simulink model "disturbances"  (R2018b)
settings: Solver=ode45  StartTime=0.0  StopTime=100  RelTol=1e-3
settings Model: Creator=Bashar  LastModifiedBy=Bashar

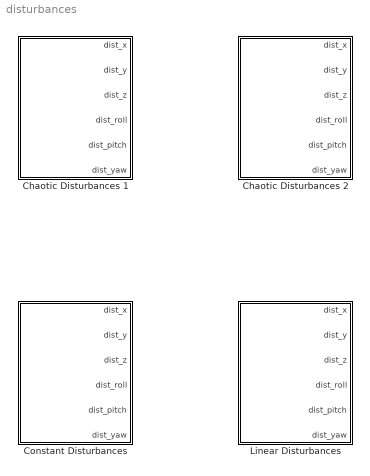
== system disturbances ==
  Chaotic Disturbances 1 : Subsystem
  Chaotic Disturbances 2 : Subsystem
  Constant Disturbances : Subsystem
  Linear Disturbances : Subsystem

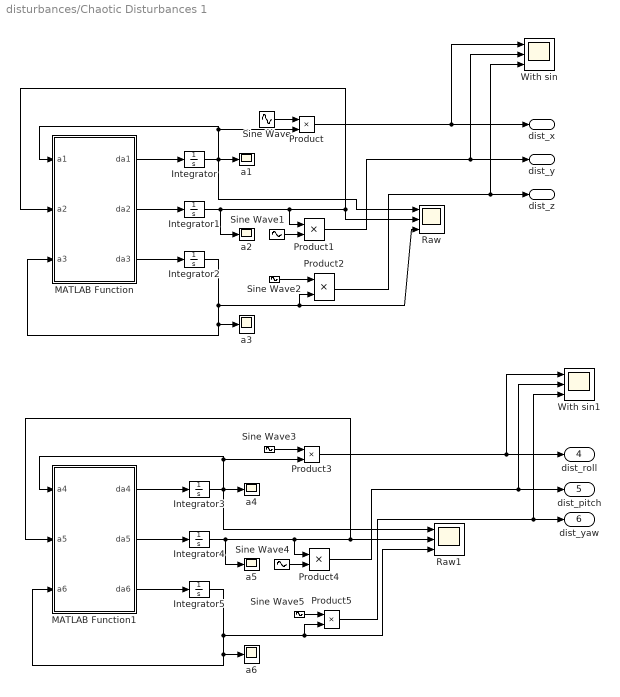
== system disturbances/Chaotic Disturbances 1 ==
  Integrator : Integrator  InitialCondition=-6
  Integrator1 : Integrator  InitialCondition=-5
  Integrator2 : Integrator  InitialCondition=22
  Integrator3 : Integrator  InitialCondition=-10
  Integrator4 : Integrator  InitialCondition=-12
  Integrator5 : Integrator  InitialCondition=24
  MATLAB Function : MATLAB Function  TreatAsAtomicUnit=on
  MATLAB Function1 : MATLAB Function  TreatAsAtomicUnit=on
  Product{,1..5} (6 alike) : Product
  Raw : Scope  NumInputPorts=3
  Raw1 : Scope  NumInputPorts=3
  Sine Wave : Sin  Amplitude=0.01  Frequency=0.5  Phase=-25  SampleTime=0
  Sine Wave1 : Sin  Amplitude=0.01  Frequency=0.5  Phase=-45  SampleTime=0
  Sine Wave2 : Sin  Amplitude=0.01  Frequency=0.5  Phase=-65  SampleTime=0
  Sine Wave3 : Sin  Amplitude=0.01  Frequency=0.5  Phase=-10  SampleTime=0
  Sine Wave4 : Sin  Amplitude=0.01  Frequency=0.5  Phase=-30  SampleTime=0
  Sine Wave5 : Sin  Amplitude=0.01  Frequency=0.5  Phase=-50  SampleTime=0
  With sin : Scope  NumInputPorts=3
  With sin1 : Scope  NumInputPorts=3
  "a1 " : Scope
  a{2..6} (5 alike) : Scope
  dist_x : Outport
  dist_y : Outport  Port=2
  dist_z : Outport  Port=3
  dist_roll : Outport  Port=4
  dist_pitch : Outport  Port=5
  dist_yaw : Outport  Port=6
  wires:
  MATLAB Function1/2(da5) -> Integrator4/1
  Sine Wave3/1 -> Product3/1
  Sine Wave4/1 -> Product4/2
  Product5/1 -> With sin1/3, dist_yaw/1
  Sine Wave5/1 -> Product5/1
  Integrator4/1 -> Product4/1, MATLAB Function1/2(a5), Raw1/2, a5/1
  Integrator/1 -> Raw/1, MATLAB Function/1(a1), Product/2, "a1 "/1
  Sine Wave/1 -> Product/1
  Integrator3/1 -> Raw1/1, MATLAB Function1/1(a4), Product3/2, a4/1
  MATLAB Function/3(da3) -> Integrator2/1
  MATLAB Function1/1(da4) -> Integrator3/1
  Product3/1 -> With sin1/1, dist_roll/1
  MATLAB Function1/3(da6) -> Integrator5/1
  Product4/1 -> With sin1/2, dist_pitch/1
  Integrator1/1 -> Product1/1, MATLAB Function/2(a2), Raw/2, a2/1
  MATLAB Function/2(da2) -> Integrator1/1
  MATLAB Function/1(da1) -> Integrator/1
  Integrator2/1 -> Product2/2, Raw/3, MATLAB Function/3(a3), a3/1
  Sine Wave2/1 -> Product2/1
  Sine Wave1/1 -> Product1/2
  Product2/1 -> With sin/3, dist_z/1
  Product/1 -> With sin/1, dist_x/1
  Product1/1 -> With sin/2, dist_y/1
  Integrator5/1 -> Product5/2, Raw1/3, MATLAB Function1/3(a6), a6/1

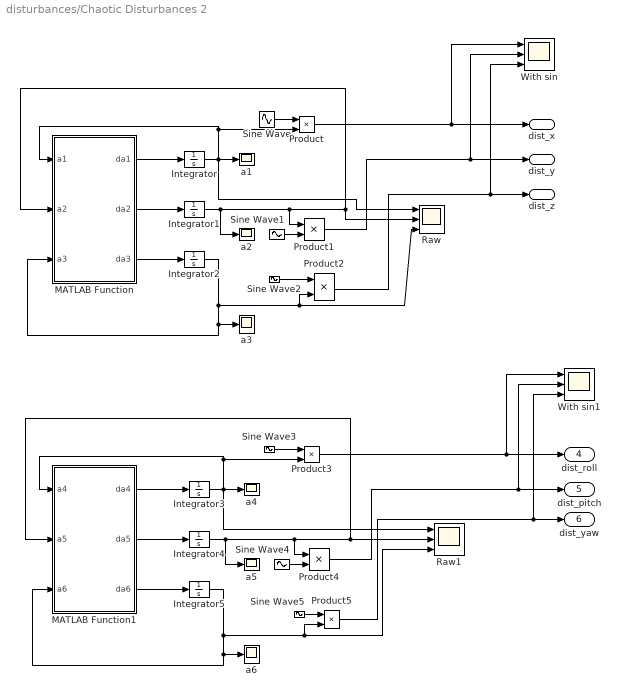
== system disturbances/Chaotic Disturbances 2 ==
  Integrator : Integrator  InitialCondition=-2
  Integrator1 : Integrator  InitialCondition=-8
  Integrator2 : Integrator  InitialCondition=15
  Integrator3 : Integrator  InitialCondition=-4
  Integrator4 : Integrator  InitialCondition=-15
  Integrator5 : Integrator  InitialCondition=20
  MATLAB Function : MATLAB Function  TreatAsAtomicUnit=on
  MATLAB Function1 : MATLAB Function  TreatAsAtomicUnit=on
  Product{,1..5} (6 alike) : Product
  Raw : Scope  NumInputPorts=3
  Raw1 : Scope  NumInputPorts=3
  Sine Wave : Sin  Amplitude=0.01  Frequency=0.5  Phase=-20  SampleTime=0
  Sine Wave1 : Sin  Amplitude=0.01  Frequency=0.5  Phase=-40  SampleTime=0
  Sine Wave2 : Sin  Amplitude=0.01  Frequency=0.5  Phase=-60  SampleTime=0
  Sine Wave3 : Sin  Amplitude=0.01  Frequency=0.5  Phase=-15  SampleTime=0
  Sine Wave4 : Sin  Amplitude=0.01  Frequency=0.5  Phase=-35  SampleTime=0
  Sine Wave5 : Sin  Amplitude=0.01  Frequency=0.5  Phase=-55  SampleTime=0
  With sin : Scope  NumInputPorts=3
  With sin1 : Scope  NumInputPorts=3
  "a1 " : Scope
  a{2..6} (5 alike) : Scope
  dist_x : Outport
  dist_y : Outport  Port=2
  dist_z : Outport  Port=3
  dist_roll : Outport  Port=4
  dist_pitch : Outport  Port=5
  dist_yaw : Outport  Port=6
  wires:
  MATLAB Function1/2(da5) -> Integrator4/1
  Sine Wave3/1 -> Product3/1
  Sine Wave4/1 -> Product4/2
  Product5/1 -> With sin1/3, dist_yaw/1
  Sine Wave5/1 -> Product5/1
  Integrator4/1 -> Product4/1, MATLAB Function1/2(a5), Raw1/2, a5/1
  Integrator/1 -> Raw/1, MATLAB Function/1(a1), Product/2, "a1 "/1
  Sine Wave/1 -> Product/1
  Integrator3/1 -> Raw1/1, MATLAB Function1/1(a4), Product3/2, a4/1
  MATLAB Function/3(da3) -> Integrator2/1
  MATLAB Function1/1(da4) -> Integrator3/1
  Product3/1 -> With sin1/1, dist_roll/1
  MATLAB Function1/3(da6) -> Integrator5/1
  Product4/1 -> With sin1/2, dist_pitch/1
  Integrator1/1 -> Product1/1, MATLAB Function/2(a2), Raw/2, a2/1
  MATLAB Function/2(da2) -> Integrator1/1
  MATLAB Function/1(da1) -> Integrator/1
  Integrator2/1 -> Product2/2, Raw/3, MATLAB Function/3(a3), a3/1
  Sine Wave2/1 -> Product2/1
  Sine Wave1/1 -> Product1/2
  Product2/1 -> With sin/3, dist_z/1
  Product/1 -> With sin/1, dist_x/1
  Product1/1 -> With sin/2, dist_y/1
  Integrator5/1 -> Product5/2, Raw1/3, MATLAB Function1/3(a6), a6/1

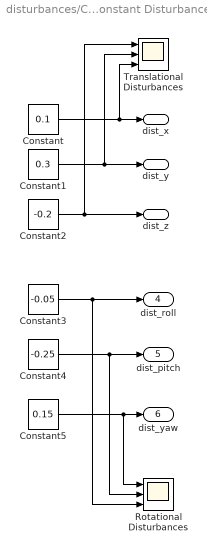
== system disturbances/Constant Disturbances ==
  Constant : Constant  Value=0.1
  Constant1 : Constant  Value=0.3
  Constant2 : Constant  Value=-0.2
  Constant3 : Constant  Value=-0.05
  Constant4 : Constant  Value=-0.25
  Constant5 : Constant  Value=0.15
  Rotational Disturbances : Scope  NumInputPorts=3
  Translational Disturbances : Scope  NumInputPorts=3
  dist_x : Outport
  dist_y : Outport  Port=2
  dist_z : Outport  Port=3
  dist_roll : Outport  Port=4
  dist_pitch : Outport  Port=5
  dist_yaw : Outport  Port=6
  wires:
  Constant/1 -> Translational Disturbances/3, dist_x/1
  Constant1/1 -> Translational Disturbances/2, dist_y/1
  Constant2/1 -> Translational Disturbances/1, dist_z/1
  Constant3/1 -> Rotational Disturbances/3, dist_roll/1
  Constant4/1 -> dist_pitch/1, Rotational Disturbances/2
  Constant5/1 -> Rotational Disturbances/1, dist_yaw/1

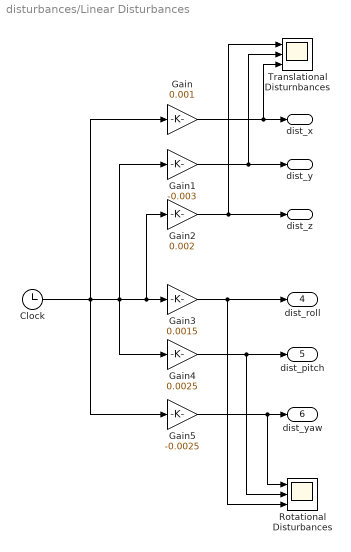
== system disturbances/Linear Disturbances ==
  Clock : Clock
  Gain : Gain  Gain=0.001
  Gain1 : Gain  Gain=-0.003
  Gain2 : Gain  Gain=0.002
  Gain3 : Gain  Gain=0.0015
  Gain4 : Gain  Gain=0.0025
  Gain5 : Gain  Gain=-0.0025
  Rotational Disturbances : Scope  NumInputPorts=3
  Translational Disturnbances : Scope  NumInputPorts=3
  dist_x : Outport
  dist_y : Outport  Port=2
  dist_z : Outport  Port=3
  dist_roll : Outport  Port=4
  dist_pitch : Outport  Port=5
  dist_yaw : Outport  Port=6
  wires:
  Gain/1 -> Translational Disturnbances/3, dist_x/1
  Gain1/1 -> Translational Disturnbances/2, dist_y/1
  Gain2/1 -> Translational Disturnbances/1, dist_z/1
  Gain3/1 -> dist_roll/1, Rotational Disturbances/3
  Gain4/1 -> dist_pitch/1, Rotational Disturbances/2
  Gain5/1 -> Rotational Disturbances/1, dist_yaw/1
  Clock/1 -> Gain2/1, Gain3/1, Gain4/1, Gain1/1, Gain5/1, Gain/1

== matlab function disturbances/Chaotic Disturbances 2/MATLAB Function ==
  data: a1 input; da1 output; a2 input; a3 input; da2 output; da3 output
function [da1, da2, da3] = lorenz_system(a1, a2, a3)
sigma = 10; rho = 28; beta = 8/3;
da1 = 0.1*(sigma*(a2-a1));
da2 = 0.1*(rho*a1 - a2 - a1*a3);
da3 = 0.1*(a1*a2 - beta*a3);
end

== matlab function disturbances/Chaotic Disturbances 2/MATLAB Function1 ==
  data: a4 input; da4 output; a5 input; a6 input; da5 output; da6 output
function [da4, da5, da6] = lorenz_system(a4, a5, a6)
sigma = 10; rho = 28; beta = 8/3;
da4 = 0.1*(sigma*(a5-a4));
da5 = 0.1*(rho*a4 - a5 - a4*a6);
da6 = 0.1*(a4*a5 - beta*a6);
end

== matlab function disturbances/Chaotic Disturbances 1/MATLAB Function ==
  data: a1 input; da1 output; a2 input; a3 input; da2 output; da3 output
function [da1, da2, da3] = lorenz_system(a1, a2, a3)
sigma = 10; rho = 28; beta = 8/3;
da1 = 0.15*(sigma*(a2-a1));
da2 = 0.15*(rho*a1 - a2 - a1*a3);
da3 = 0.15*(a1*a2 - beta*a3);
end

== matlab function disturbances/Chaotic Disturbances 1/MATLAB Function1 ==
  data: a4 input; da4 output; a5 input; a6 input; da5 output; da6 output
function [da4, da5, da6] = lorenz_system(a4, a5, a6)
sigma = 10; rho = 28; beta = 8/3;
da4 = 0.15*(sigma*(a5-a4));
da5 = 0.15*(rho*a4 - a5 - a4*a6);
da6 = 0.15*(a4*a5 - beta*a6);
end
